simulink model "Ex2"  (R2019b)
settings: Solver=VariableStepAuto  StartTime=0.0  StopTime=50.0  RelTol=1e-3
settings Model: Creator=ovi  LastModifiedBy=ovi

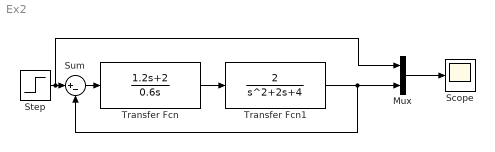
== system Ex2 ==
  Mux : Mux  Inputs=2
  Scope : Scope
  Step : Step  SampleTime=0
  Sum : Sum  Inputs=|+-
  Transfer Fcn : TransferFcn  Numerator=[1.2 2]  Denominator=[0.6 0]
  Transfer Fcn1 : TransferFcn  Numerator=2  Denominator=[1 2 4]
  wires:
  Mux/1 -> Scope/1
  Transfer Fcn/1 -> Transfer Fcn1/1
  Step/1 -> Sum/1, Mux/1
  Transfer Fcn1/1 -> Sum/2, Mux/2
  Sum/1 -> Transfer Fcn/1
